simulink model "H_Bridge_Control"  (R2025a)
settings: Solver=FixedStepAuto  StartTime=0.0  StopTime=inf  RelTol=1e-3  EnableMultiTasking=on
undefined symbols (not defined in the file): DiscIntNeverNeededParam
libraries: stm32f4xxblockslib x2, stm32g4xxblockslib x1, stm32blockslib x1
settings Model: STM32="{\"AnalogInput\":{\"ID\":\"H_Bridge_Control:1\"},\"HRTimer\":{\"ID\":\"H_Bridge_Control:2\"},\"HardwareInterrupt\":{\"ID\":\"H_Bridge_Control:3\"},\"DigitalPortWrite\":{\"ID\":\"H_Bridge_Control:42\"}}"  Creator=GNKRISHNAN  LastModifiedBy=GNKRISHNAN
settings SolverCC: AutoInsertRateTranBlk=on
settings OptimizationCC: DefaultParameterBehavior=Inlined  EnhancedBackFolding=on  PassReuseOutputArgsAs=Individual arguments  ZeroExternalMemoryAtStartup=off  ZeroInternalMemoryAtStartup=off  MaxStackSize=512  OptimizeBlockOrder=speed  DifferentSizesBufferReuse=on  OptimizationCustomize=off  EfficientTunableParamExpr=on
settings DebuggingCC: ParameterTunabilityLossMsg=error
settings HardwareCC: ProdBitPerPointer=32.0  ProdBitPerSizeT=32.0  ProdBitPerPtrDiffT=32.0  ProdLargestAtomicInteger=Long  ProdLargestAtomicFloat=Double  ProdWordSize=32.0  ProdLongLongMode=on  ProdHWDeviceType=ARM Compatible->ARM Cortex-M
settings SFSimCC: MATLABDynamicMemAlloc=off
settings RTWCC: SystemTargetFile=ert.tlc  HardwareBoard=STM32G4xx Based  TemplateMakefile=ert_default_tmf  Toolchain=GNU Tools for ARM Embedded Processors  Description=Embedded Coder
settings CodeAppCC: ForceParamTrailComments=on  IgnoreCustomStorageClasses=off  OperatorAnnotations=on  SimulinkDataObjDesc=on  SFDataObjDesc=on  InsertBlockDesc=on
settings ERTTargetCC: ExtModeTransport=3.0  ExtModeStaticAllocSize=2048.0  TargetLangStandard=C99 (ISO)  CodeReplacementLibrary=ARM Cortex-M

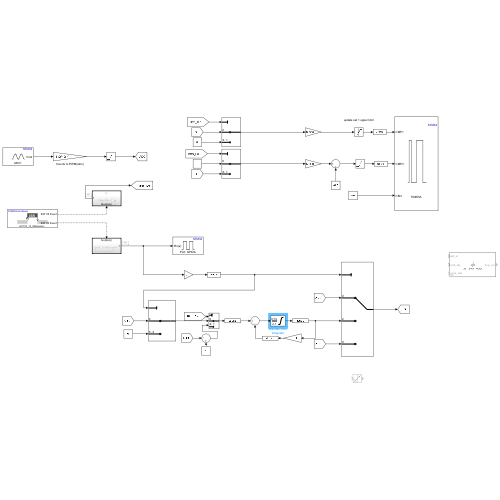
[thumbnail: Simulink's stored preview of the top-level diagram]
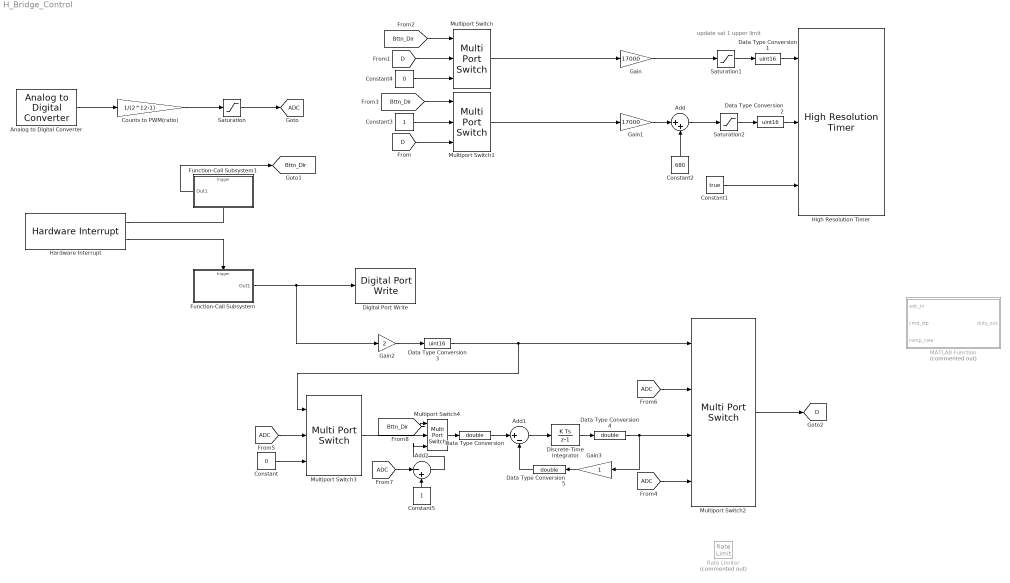
== system H_Bridge_Control ==
  note: update sat 1 upper limit
  Add : Sum  Inputs=|++
  Add1 : Sum  Inputs=|+-
  Add2 : Sum  Inputs=|-+
  Analog to Digital Converter : stm32f4xxblockslib/Analog to Digital Converter  ADCModule=ADC1  ConversionGroup=Regular  TriggerMode=Trigger and read  NumberOfConversions=1  EnableBufferConv=off  BufferLength=1  OutputStatus=off  SampleTime=-1  EnableSimPort=off  hoistedMaskSrc=ECSoC/ECSimCodegen/Analog to Digital Converter
  Constant : Constant  Value=0
  Constant1 : Constant  Value=true
  Constant2 : Constant  Value=680
  Constant3 : Constant
  Constant4 : Constant  Value=0
  Constant5 : Constant
  Counts to PWM(ratio) : Gain  Gain=1/(2^12-1)
  Data Type Conversion : DataTypeConversion  OutDataTypeStr=double  SaturateOnIntegerOverflow=off  RndMeth=Floor
  Data Type Conversion1 : DataTypeConversion  OutDataTypeStr=uint16  SaturateOnIntegerOverflow=off  RndMeth=Floor
  Data Type Conversion2 : DataTypeConversion  OutDataTypeStr=uint16  SaturateOnIntegerOverflow=off  RndMeth=Floor
  Data Type Conversion3 : DataTypeConversion  OutDataTypeStr=uint16  SaturateOnIntegerOverflow=off  RndMeth=Floor
  Data Type Conversion4 : DataTypeConversion  OutDataTypeStr=double  SaturateOnIntegerOverflow=off  RndMeth=Floor
  Data Type Conversion5 : DataTypeConversion  OutDataTypeStr=double  SaturateOnIntegerOverflow=off  RndMeth=Floor
  Digital Port Write : stm32f4xxblockslib/Digital Port Write  PortName=GPIOA  PinNumber=[5]  ReadOperation=off  IOAsArray=on  EnableSimPort=off  hoistedMaskSrc=ECSoC/ECSimCodegen/Digital Port Write
      settings: LibrarySourceBlock=stm32g4xxblockslib/Digital Port Write
  Discrete-Time Integrator : DiscreteIntegrator  gainval=1.5  SampleTime=-1  LimitOutput=on  UpperSaturationLimit=1.0  LowerSaturationLimit=0.0  ICPrevOutput=DiscIntNeverNeededParam  ICPrevScaledInput=DiscIntNeverNeededParam
  Function-Call Subsystem : Subsystem  TreatAsAtomicUnit=on
  Function-Call Subsystem1 : Subsystem  TreatAsAtomicUnit=on
  Gain : Gain  Gain=17000
  Gain1 : Gain  Gain=17000
  Gain2 : Gain  Gain=2
  Gain3 : Gain
  Hardware Interrupt : stm32g4xxblockslib/Hardware Interrupt  ISRGroup=External interrupts (EXTI)  ISRName=EXTI15_10_IRQHandler  ISRNumber=55  EventsList={ 'on', 'EXTI15 Event', '1'; 'off', 'EXTI14 Event', '2'; 'on', 'EXTI13 Event', '3'; 'off', 'EXTI12 Event', '4'; 'off', 'EXTI11 Event', '5'; 'off', 'EXTI10 Event', '6'; 'off', 'Custom event', '7' }  SelectedEvents={'EXTI15 Event','EXTI13 Event'}  TaskPriority=30  DisablePreemption=off  ClearInterruptFlagsAtEndOfEvent=off  InterruptDefinitionFile=$(TARGET_ROOT)/registry/interrupts/STM32F4xxBased_interrupts.xml  HardwareBoard=STM32G4xx Based  EnableSimPort=off
  High Resolution Timer : stm32blockslib/High Resolution Timer  TimerModule=TIMERA  EnableChannel1=on  EnableChannel2=on  EnableFrequencyInput=off  EnableCounterStartStopInput=on  Channel1DisableStatus=off  Channel2DisableStatus=off  EnableDLLcalibation=off  SampleTime=-1  CMPUnits=Counts  CMP1Input=on  CMP2Input=off  CMP3Input=on  CMP4Input=off  EnableUpdateEvent=off  Channel1activeState=off  Channel2activeState=off  Channel1InactiveState=off  Channel2InactiveState=off
      settings: LibrarySourceBlock=stm32g4xxblockslib/High Resolution Timer
  MATLAB Function : MATLAB Function  Commented=on  TreatAsAtomicUnit=on
  Multiport Switch : MultiPortSwitch  DataPortOrder=Zero-based contiguous  Inputs=2  zeroidx=on  SaturateOnIntegerOverflow=off  InputSameDT=off
  Multiport Switch1 : MultiPortSwitch  DataPortOrder=Zero-based contiguous  Inputs=2  zeroidx=on  SaturateOnIntegerOverflow=off  InputSameDT=off
  Multiport Switch2 : MultiPortSwitch  DataPortOrder=Specify indices  DataPortIndices={0,2}  DataPortForDefault=Additional data port  SaturateOnIntegerOverflow=off  InputSameDT=off
  Multiport Switch3 : MultiPortSwitch  DataPortOrder=Specify indices  DataPortIndices={0,2}  SaturateOnIntegerOverflow=off  InputSameDT=off
  Multiport Switch4 : MultiPortSwitch  DataPortOrder=Specify indices  DataPortIndices={0,1}  SaturateOnIntegerOverflow=off  InputSameDT=off
  Rate Limiter : RateLimiter  Commented=on  RisingSlewLimit=0.1  FallingSlewLimit=-0.1  SampleTimeMode=inherited
  Saturation : Saturate  UpperLimit=1  LowerLimit=0
  Saturation1 : Saturate  UpperLimit=15640  LowerLimit=0
  Saturation2 : Saturate  UpperLimit=16319  LowerLimit=680
  tag scope: ADC=global, Bttn_Dir=global, D=global
  wires:
  Analog to Digital Converter/1 -> Counts to PWM(ratio)/1
  Hardware Interrupt/2 -> Function-Call Subsystem/Trigger
  Gain1/1 -> Add/1
  Add/1 -> Saturation2/1
  Constant2/1 -> Add/2
  Gain/1 -> Saturation1/1
  Constant1/1 -> High Resolution Timer/3
  Saturation1/1 -> Data Type Conversion1/1
  Saturation2/1 -> Data Type Conversion2/1
  Data Type Conversion1/1 -> High Resolution Timer/1
  Data Type Conversion2/1 -> High Resolution Timer/2
  Function-Call Subsystem/1(Out1) -> Gain2/1, Digital Port Write/1
  Hardware Interrupt/1 -> Function-Call Subsystem1/Trigger
  Counts to PWM(ratio)/1 -> Saturation/1
  Function-Call Subsystem1/1(Out1) -> [Bttn_Dir]
  Saturation/1 -> [ADC]
  Multiport Switch/1 -> Gain/1
  Constant3/1 -> Multiport Switch1/2
  Constant4/1 -> Multiport Switch/3
  [D] -> Multiport Switch/2
  Multiport Switch1/1 -> Gain1/1
  [D] -> Multiport Switch1/3
  [Bttn_Dir] -> Multiport Switch/1
  [Bttn_Dir] -> Multiport Switch1/1
  Gain2/1 -> Data Type Conversion3/1
  [ADC] -> Multiport Switch2/2
  Data Type Conversion3/1 -> Multiport Switch3/1, Multiport Switch2/1
  [ADC] -> Multiport Switch2/4
  Multiport Switch2/1 -> [D]
  Add1/1 -> Discrete-Time Integrator/1
  Discrete-Time Integrator/1 -> Data Type Conversion4/1
  Data Type Conversion5/1 -> Add1/2
  Gain3/1 -> Data Type Conversion5/1
  Constant/1 -> Multiport Switch3/3
  [ADC] -> Multiport Switch3/2
  Multiport Switch3/1 -> Multiport Switch4/2
  Data Type Conversion4/1 -> Gain3/1, Multiport Switch2/3
  Data Type Conversion/1 -> Add1/1
  Multiport Switch4/1 -> Data Type Conversion/1
  [ADC] -> Add2/1
  Add2/1 -> Multiport Switch4/3
  Constant5/1 -> Add2/2
  [Bttn_Dir] -> Multiport Switch4/1

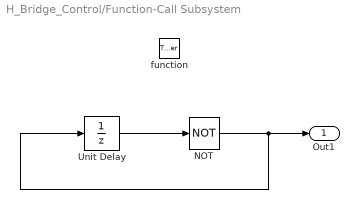
== system H_Bridge_Control/Function-Call Subsystem ==
  function : TriggerPort  TriggerType=function-call  VariantControl=(inherit)
  NOT : Logic  Operator=NOT  IconShape=distinctive  AllPortsSameDT=off  OutDataTypeStr=boolean
  Unit Delay : UnitDelay  InitialCondition=1  SampleTime=-1  HasFrameUpgradeWarning=on
  Out1 : Outport
  wires:
  NOT/1 -> Unit Delay/1, Out1/1
  Unit Delay/1 -> NOT/1

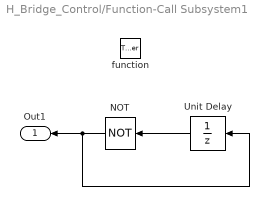
== system H_Bridge_Control/Function-Call Subsystem1 ==
  function : TriggerPort  TriggerType=function-call  VariantControl=(inherit)
  NOT : Logic  Operator=NOT  IconShape=distinctive  AllPortsSameDT=off  OutDataTypeStr=boolean
  Unit Delay : UnitDelay  SampleTime=-1  HasFrameUpgradeWarning=on
  Out1 : Outport
  wires:
  NOT/1 -> Unit Delay/1, Out1/1
  Unit Delay/1 -> NOT/1

== matlab function H_Bridge_Control/MATLAB Function ==
  data: adc_in input; duty_out output; cmd_stp input; ramp_rate input
function duty_out = fcn_stop_ramp(adc_in, cmd_stp, ramp_rate)
%#codegen

persistent duty_cur
if isempty(duty_cur)
    duty_cur = single(0.0);
end

step        = single(ramp_rate);
setpoint    = min(max(single(adc_in), single(0.0)), single(1.0));
stop_active = (double(cmd_stp) == 2.0);

if stop_active
    duty_cur = max(duty_cur - step, single(0.0));
else
    if duty_cur < setpoint
        duty_cur = min(duty_cur + step, setpoint);
    elseif duty_cur > setpoint
        duty_cur = max(duty_cur - step, setpoint);
    end
end

duty_out = duty_cur;
end
